simulink model "prob3"  (R2020b)
settings: Solver=VariableStepAuto  StartTime=0.0  StopTime=10.0  RelTol=1e-3
settings Model: Creator=stkaravind  LastModifiedBy=stkaravind

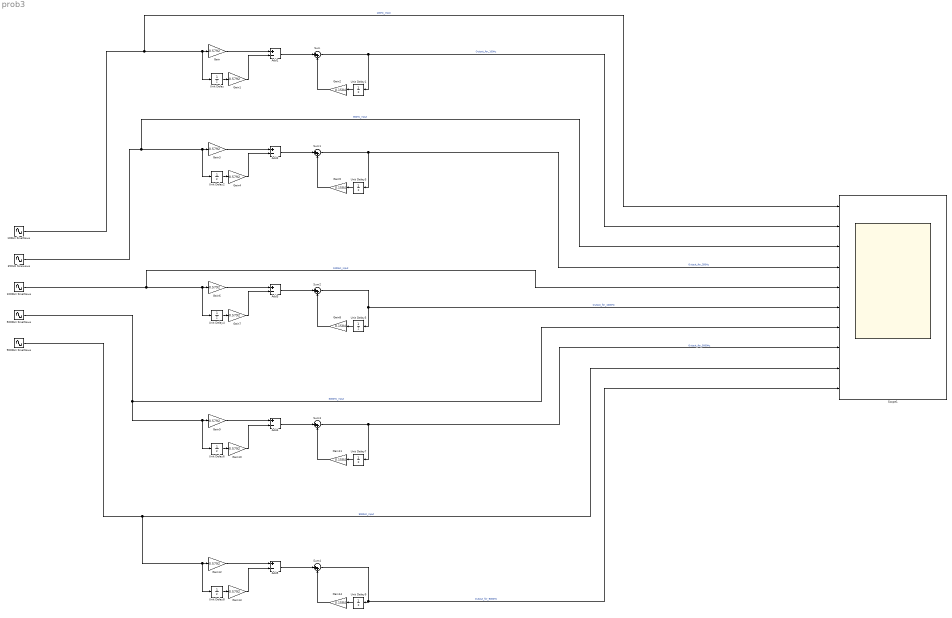
== system prob3 ==
  1000Hz SineWave : Sin  Frequency=2*pi*1000  SampleTime=0
  100Hz SineWave : Sin  Frequency=2*pi*100  SampleTime=0
  350Hz Sinewave : Sin  Frequency=2*pi*350  SampleTime=0
  5000Hz SineWave : Sin  Frequency=2*pi*5000  SampleTime=0
  9000Hz SineWave : Sin  Frequency=2*pi*9000  SampleTime=0
  Add{1..5} (5 alike) : Sum  Inputs=+-
  Gain{,1,3..4,6..7,9..10,12..13} (10 alike) : Gain  Gain=0.5792
  Gain{2,5,8,11,14} (5 alike) : Gain  Gain=0.1584
  Scope1 : Scope  NumInputPorts=10
  Sum{,1..4} (5 alike) : Sum  Inputs=|++
  Unit Delay{,1..9} (10 alike) : UnitDelay  SampleTime=-1  HasFrameUpgradeWarning=on
  wires:
  Add1/1 -> Sum/1
  Sum/1 -> Scope1/2, Unit Delay1/1  "Output_for_100Hz"
  Gain6/1 -> Add3/1
  Add3/1 -> Sum2/1
  350Hz Sinewave/1 -> Scope1/3, Unit Delay2/1, Gain3/1  "350Hz_Input"
  Add2/1 -> Sum1/1
  Gain14/1 -> Sum4/2
  5000Hz SineWave/1 -> Unit Delay6/1, Gain9/1, Scope1/7  "5000Hz_Input"
  Gain/1 -> Add1/1
  Gain2/1 -> Sum/2
  Sum1/1 -> Unit Delay3/1, Scope1/4  "Output_for_350Hz"
  1000Hz SineWave/1 -> Scope1/5, Unit Delay4/1, Gain6/1  "1000Hz_Input"
  Unit Delay/1 -> Gain1/1
  Add5/1 -> Sum4/1
  Unit Delay5/1 -> Gain8/1
  Gain3/1 -> Add2/1
  Unit Delay3/1 -> Gain5/1
  Gain1/1 -> Add1/2
  Unit Delay2/1 -> Gain4/1
  Sum2/1 -> Unit Delay5/1, Scope1/6  "Output_for_1000Hz"
  Gain5/1 -> Sum1/2
  Unit Delay8/1 -> Gain13/1
  100Hz SineWave/1 -> Scope1/1, Unit Delay/1, Gain/1  "100Hz_Input"
  Unit Delay6/1 -> Gain10/1
  Gain9/1 -> Add4/1
  Gain12/1 -> Add5/1
  Gain7/1 -> Add3/2
  Gain11/1 -> Sum3/2
  Gain8/1 -> Sum2/2
  Unit Delay7/1 -> Gain11/1
  Gain10/1 -> Add4/2
  9000Hz SineWave/1 -> Unit Delay8/1, Gain12/1, Scope1/9  "9000Hz_Input"
  Unit Delay9/1 -> Gain14/1
  Unit Delay4/1 -> Gain7/1
  Add4/1 -> Sum3/1
  Sum4/1 -> Unit Delay9/1, Scope1/10  "Output_for_9000Hz"
  Gain4/1 -> Add2/2
  Unit Delay1/1 -> Gain2/1
  Gain13/1 -> Add5/2
  Sum3/1 -> Unit Delay7/1, Scope1/8  "Output_for_5000Hz"
